simulink model "mpcVehicleSteering"  (R2017b)
settings: Solver=VariableStepAuto  StartTime=0.0  StopTime=15  RelTol=1e-3
values from neighbouring files (symbols this model uses):
  Ts = 0.1    [VehicleSteeringControlExample.m]    (also in run_Leader_follower.m; run_ParetoBlending.m; run_ParetoSwitching.m)
  Vx = 10    [RandomizedBlending.m]    (also in VehicleSteeringControlExample.m = 15; run_Leader_follower.m; run_ParetoBlending.m; run_ParetoSwitching.m)
libraries: mpclib x2, cstblocks x1
settings Model: Creator=The MathWorks, Inc.  LastModifiedBy=Yves
settings CodeAppCC: StateflowObjectComments=on
settings SimscapeCC: SimscapeNormalizeSystem=off

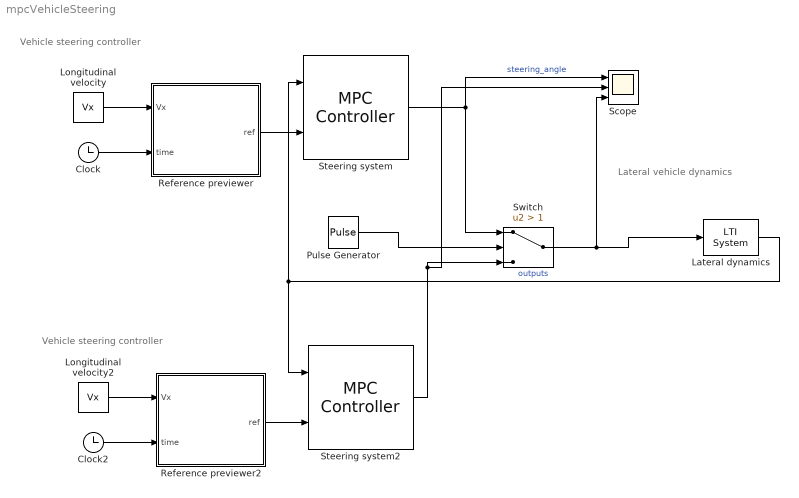
== system mpcVehicleSteering ==
  note: Lateral vehicle dynamics
  note: Vehicle steering controller
  note: Vehicle steering controller
  Clock : Clock
  Clock2 : Clock
  Lateral dynamics : cstblocks/LTI System  sys=vehicle  IC=[]
  Longitudinal velocity : Constant  Value=Vx  SampleTime=Ts
  Longitudinal velocity2 : Constant  Value=Vx  SampleTime=Ts
  Pulse Generator : DiscretePulseGenerator  PulseType=Time based  Amplitude=2  Period=1  PulseWidth=50
  Reference previewer : MATLAB Function  TreatAsAtomicUnit=on  SystemSampleTime=Ts
  Reference previewer2 : MATLAB Function  TreatAsAtomicUnit=on  SystemSampleTime=Ts
  Scope : Scope  NumInputPorts=3
  Steering system : mpclib/MPC Controller  SCDEnableBlockLinearizationSpecification=on  mpcobj=mpc1  is_multiple=0  enable_value=0  return_u0=off  ref_from_ws=off  ref_signal_name=[]  ref_preview=off  md_from_ws=off  md_signal_name=[]  md_preview=off  from_project=off  project_file=MPCtask.mat  md_inport=off  mv_inport=off  cost_outport=off  return_sequence=off  return_qpstatus=off  return_state=off  state_inport=off  lims_inport=off  cc_inport=off  ywt_inport=off  is_designfromscratch=0  uwt_inport=off  duwt_inport=off  rhoeps_inport=off  uref_inport=off  n_ts=0.1  n_p=10  n_mv=1  n_md=0  n_ud=0  n_mo=2  n_uo=0  BlockDataType=double  SampleTimeInherited=off  switch_inport=off
  Steering system2 : mpclib/MPC Controller  SCDEnableBlockLinearizationSpecification=on  mpcobj=HumanMPC  is_multiple=0  enable_value=0  return_u0=off  ref_from_ws=off  ref_signal_name=[]  ref_preview=off  md_from_ws=off  md_signal_name=[]  md_preview=off  from_project=off  project_file=MPCtask.mat  md_inport=off  mv_inport=off  cost_outport=off  return_sequence=off  return_qpstatus=off  return_state=off  state_inport=off  lims_inport=off  cc_inport=off  ywt_inport=off  is_designfromscratch=0  uwt_inport=off  duwt_inport=off  rhoeps_inport=off  uref_inport=off  n_ts=0.1  n_p=10  n_mv=1  n_md=0  n_ud=0  n_mo=2  n_uo=0  BlockDataType=double  SampleTimeInherited=off  switch_inport=off
  Switch : Switch  Criteria=u2 > Threshold  Threshold=1
  wires:
  Longitudinal velocity/1 -> Reference previewer/1(Vx)
  Steering system/1 -> Scope/1, Switch/1  "steering_angle"
  Clock/1 -> Reference previewer/2(time)
  Reference previewer/1(ref) -> Steering system/2
  Lateral dynamics/1 -> Steering system/1, Steering system2/1  "outputs"
  Pulse Generator/1 -> Switch/2
  Steering system2/1 -> Scope/2, Switch/3
  Switch/1 -> Scope/3, Lateral dynamics/1
  Reference previewer2/1(ref) -> Steering system2/2
  Longitudinal velocity2/1 -> Reference previewer2/1(Vx)
  Clock2/1 -> Reference previewer2/2(time)

== matlab function mpcVehicleSteering/Reference previewer ==
  data: Vx input; time input; ref output
function ref = previewer(Vx,time)
% Get previewed reference trajectory

% Previw horizon is 10 sampling times (i.e. 10*0.1 = 1 seconds).
% Reference contains 2 signals (i.e. Y position and yaw angle).
ref = zeros(10,2); 

%% Previewing sequence
for ct = 1:10
   ref(ct,:) = doubleLaneChange(Vx,time + (ct-1)*0.1);
end

== matlab function mpcVehicleSteering/Reference previewer2 ==
  data: Vx input; time input; ref output
function ref = previewer(Vx,time)
% Get previewed reference trajectory

% Previw horizon is 10 sampling times (i.e. 10*0.1 = 1 seconds).
% Reference contains 2 signals (i.e. Y position and yaw angle).
ref = zeros(10,2); 

%% Previewing sequence
for ct = 1:10
   ref(ct,:) = doubleLaneChange(Vx,time + (ct-1)*0.1);
end
